simulink model "Sim1_4"  (R2017a)
settings: Solver=ode45  StartTime=tstart  StopTime=tstop  RelTol=1e-3  EnableMultiTasking=on
values from neighbouring files (symbols this model uses):
  c = 0    [run_task_1_2.m]    (also in run_task_1_3.m = 1; run_task_1_4.m; run_task_1_6.m; run_task_1_8.m)
  K_d = -K_d    [run_task_1_3.m]    (also in run_task_1_8.m = 350)
  K_i = 0*K_p*omega_n/10    [run_task_1_3.m]    (also in run_task_1_8.m = 0)
  K_p = (m+K_m)*omega_n^2-k    [run_task_1_3.m]    (also in run_task_1_8.m = -18)
  psi0 = 0    [run_task_1_2.m]    (also in run_task_1_3.m; run_task_1_4.m; run_task_1_6.m; run_task_1_8.m)
  r0 = 0    [run_task_1_2.m]    (also in run_task_1_3.m; run_task_1_4.m; run_task_1_6.m; run_task_1_8.m)
  tsamp = 10    [run_task_1_2.m]    (also in run_task_1_3.m; run_task_1_4.m; run_task_1_6.m; run_task_1_8.m)
  v0 = [4.9 0]'    [run_task_1_2.m]    (also in run_task_1_3.m = [6.63 0]'; run_task_1_4.m = [6.63 0]'; run_task_1_6.m = [0.01 0]'; run_task_1_8.m = [4 0]')
undefined symbols (not defined in the file or in its folder): msfartoystyring
undefined symbols (not defined in the file): p0
libraries: simulink x1
settings Model: ExtModeAutoUpdateStatusClock=off  Creator=christh  LastModifiedBy=Alex
settings DataIOCC: LimitDataPoints=on  SaveFormat=Array  SignalLoggingSaveFormat=ModelDataLogs
settings OptimizationCC: ExpressionDepthLimit=2147483647  InitFltsAndDblsToZero=on  LifeSpan=inf
settings DebuggingCC: UnderspecifiedInitializationDetection=Classic  MergeDetectMultiDrivingBlocksExec=none  SolverPrmCheckMsg=warning  FcnCallInpInsideContextMsg=warning  StateNameClashWarn=warning  SFUnexpectedBacktrackingDiag=warning  SFNoUnconditionalDefaultTransitionDiag=warning  SFExecutionAtInitializationDiag=none
settings HardwareCC: ProdBitPerPointer=32  ProdBitPerSizeT=32  ProdBitPerPtrDiffT=32  ProdLargestAtomicFloat=None  ProdIntDivRoundTo=Undefined  ProdEndianess=Unspecified  ProdWordSize=32  ProdHWDeviceType=32-bit Generic
settings ModelReferenceCC: PropagateSignalLabelsOutOfModel=off
settings GRTTargetCC: TargetLangStandard=C89/C90 (ANSI)  GeneratePreprocessorConditionals=Disable all  CombineOutputUpdateFcns=off  GRTInterface=on
settings ConfigComp: CovMetricSettings=dw  CovHtmlReporting=on  CovSaveCumulativeToWorkspaceVar=on  CovSaveSingleToWorkspaceVar=on  CovExternalEMLEnable=off

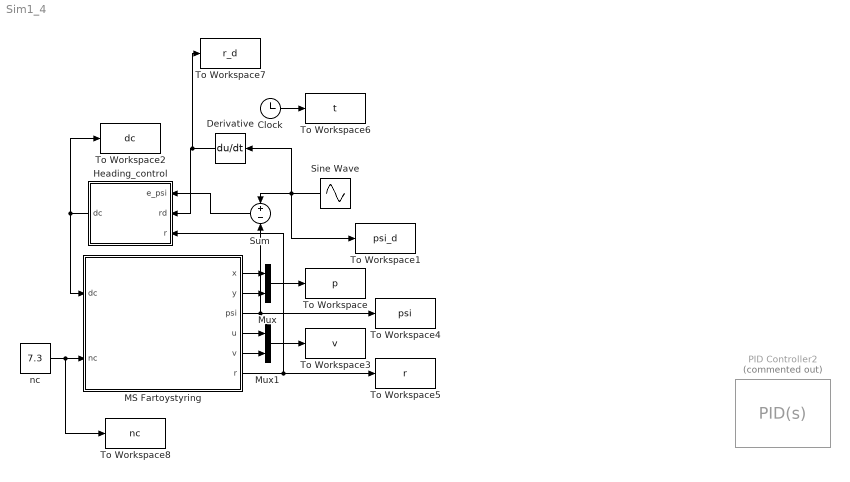
== system Sim1_4 ==
  Clock : Clock
  Derivative : Derivative
  Heading_control : Subsystem
  MS Fartoystyring : Subsystem  mask(MS Fartoystyring for Assignment 3 G&C){x0=p0(1), y0=p0(2), u0=v0(1), v0=v0(2), psi0=psi0, r0=r0, c=c}
      mask prompts: x0 "x(t0) (m)"; y0 "y(t0) (m)"; u0 "u(t0) (m/s)"; v0 "v(t0) (m/s)"; psi0 "psi(t0) (rad)"; r0 "r(t0) (rad/s)"; c "current (0 or 1)"
      mask help:
      | Block corresponding to Figure 1 in the assignment text. Gives the response of the ship.
      |
      | The design speed of MS Fartoystyring is u=8.23 m/s.
      |
      | Input:
      | dc: commanded rudder (rad), dmax=25*pi/180
      | nc: commanded shaft speed (rad/s), nmax=85*2*pi/60
      |
      | Output:
      | x: north pos (m)
      | y: east pos (m)
      | u: surge (m/s)
      | v: sway (m/s)
      | psi: heading (rad)
      | r: yaw (rad/s)
      mask Help: Comments, bugs and help requests can be directed to the TA. Email on course website.
  Mux : Mux  Inputs=2
  Mux1 : Mux  Inputs=2
  PID Controller2 : simulink/Continuous/PID Controller  Commented=on  Controller=PID  TimeDomain=Continuous-time  SampleTime=-1  IntegratorMethod=Forward Euler  FilterMethod=Forward Euler  Form=Parallel  UseFilter=on  ControllerParametersSource=internal  P=K_p  I=0  D=K_d  N=1  InitialConditionSource=internal  InitialConditionForIntegrator=0  InitialConditionForFilter=0  ExternalReset=none  LimitOutput=off  UpperSaturationLimit=inf  LowerSaturationLimit=-inf  LinearizeAsGain=on  AntiWindupMode=none  Kb=1  TrackingMode=off  Kt=1  PParamMin=[]  PParamMax=[]  IParamMin=[]  IParamMax=[]  DParamMin=[]  DParamMax=[]  NParamMin=[]  NParamMax=[]  KbParamMin=[]  KbParamMax=[]  KtParamMin=[]  KtParamMax=[]  POutMin=[]  POutMax=[]  IOutMin=[]  IOutMax=[]  DOutMin=[]  DOutMax=[]  NOutMin=[]  NOutMax=[]  KbOutMin=[]  KbOutMax=[]  KtOutMin=[]  KtOutMax=[]  IntegratorOutMin=[]  IntegratorOutMax=[]  FilterOutMin=[]  FilterOutMax=[]  SumOutMin=[]  SumOutMax=[]  SumI1OutMin=[]  SumI1OutMax=[]  SumI2OutMin=[]  SumI2OutMax=[]  SumI3OutMin=[]  SumI3OutMax=[]  SumDOutMin=[]  SumDOutMax=[]  SaturationOutMin=[]  SaturationOutMax=[]  IntegratorContinuousStateAttributes=''  IntegratorStateMustResolveToSignalObject=off  IntegratorRTWStateStorageClass=Auto  FilterContinuousStateAttributes=''  FilterStateMustResolveToSignalObject=off  FilterRTWStateStorageClass=Auto  DifferentiatorICPrevScaledInput=0  DifferentiatorOutMin=[]  DifferentiatorOutMax=[]  InitialConditionSetting=State (most efficient)
  Sine Wave : Sin  Amplitude=-0.3  Frequency=0.008  SampleTime=0
  Sum : Sum  Inputs=+-
  To Workspace : ToWorkspace  VariableName=p  SampleTime=tsamp
  To Workspace1 : ToWorkspace  VariableName=psi_d  SampleTime=tsamp
  To Workspace2 : ToWorkspace  VariableName=dc  SampleTime=tsamp
  To Workspace3 : ToWorkspace  VariableName=v  SampleTime=tsamp
  To Workspace4 : ToWorkspace  VariableName=psi  SampleTime=tsamp
  To Workspace5 : ToWorkspace  VariableName=r  SampleTime=tsamp
  To Workspace6 : ToWorkspace  VariableName=t  SampleTime=tsamp
  To Workspace7 : ToWorkspace  VariableName=r_d  SampleTime=tsamp
  To Workspace8 : ToWorkspace  VariableName=nc  SampleTime=tsamp
  nc : Constant  Value=7.3
  wires:
  MS Fartoystyring/3(psi) -> To Workspace4/1, Sum/2
  MS Fartoystyring/4(u) -> Mux1/1
  Mux/1 -> To Workspace/1
  Clock/1 -> To Workspace6/1
  Sine Wave/1 -> Derivative/1, To Workspace1/1, Sum/1
  Mux1/1 -> To Workspace3/1
  MS Fartoystyring/1(x) -> Mux/1
  MS Fartoystyring/5(v) -> Mux1/2
  MS Fartoystyring/2(y) -> Mux/2
  MS Fartoystyring/6(r) -> Heading_control/3(r), To Workspace5/1
  Heading_control/1(dc) -> To Workspace2/1, MS Fartoystyring/1(dc)
  Sum/1 -> Heading_control/1(e_psi)
  Derivative/1 -> To Workspace7/1, Heading_control/2(rd)
  nc/1 -> To Workspace8/1, MS Fartoystyring/2(nc)

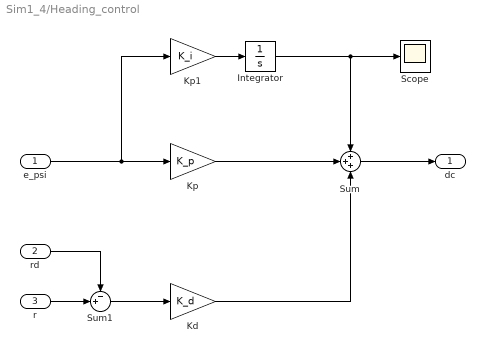
== system Sim1_4/Heading_control ==
  e_psi : Inport
  rd : Inport  Port=2
  r : Inport  Port=3
  Integrator : Integrator
  Kd : Gain  Gain=K_d
  Kp : Gain  Gain=K_p
  Kp1 : Gain  Gain=K_i
  Scope : Scope
  Sum : Sum  Inputs=+++
  Sum1 : Sum  Inputs=-+|
  dc : Outport
  wires:
  Sum/1 -> dc/1
  e_psi/1 -> Kp1/1, Kp/1
  Kp/1 -> Sum/2
  Kd/1 -> Sum/3
  Kp1/1 -> Integrator/1
  Integrator/1 -> Scope/1, Sum/1
  r/1 -> Sum1/2
  rd/1 -> Sum1/1
  Sum1/1 -> Kd/1

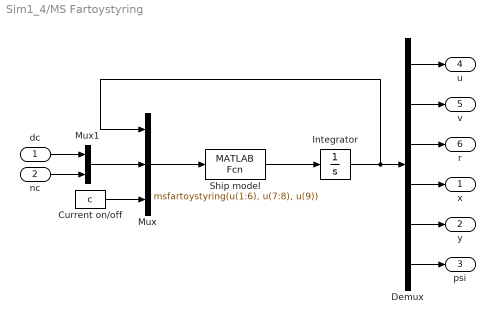
== system Sim1_4/MS Fartoystyring ==
  dc : Inport
  nc : Inport  Port=2
  Current on/off : Constant  Value=c
  Demux : Demux  Outputs=6
  Integrator : Integrator  InitialCondition=[u0 v0 r0 x0 y0 psi0]'
  Mux : Mux  Inputs=3
  Mux1 : Mux  Inputs=2
  Ship model : MATLABFcn  MATLABFcn=msfartoystyring(u(1:6), u(7:8), u(9))  OutputDimensions=6
  x : Outport
  y : Outport  Port=2
  psi : Outport  Port=3
  u : Outport  Port=4
  v : Outport  Port=5
  r : Outport  Port=6
  wires:
  Integrator/1 -> Mux/1, Demux/1
  Mux1/1 -> Mux/2
  dc/1 -> Mux1/1
  nc/1 -> Mux1/2
  Demux/1 -> u/1
  Demux/2 -> v/1
  Demux/3 -> r/1
  Demux/4 -> x/1
  Demux/5 -> y/1
  Demux/6 -> psi/1
  Current on/off/1 -> Mux/3
  Ship model/1 -> Integrator/1
  Mux/1 -> Ship model/1
